simulink model "LQG_Con_lac_nguoc"  (R2023a)
settings: Solver=FixedStepAuto  StartTime=0.0  StopTime=6  FixedStep=0.01  RelTol=1e-3
values from neighbouring files (symbols this model uses):
  A = [ 0,                                                                                                                                                                                                                                                       1,                                                                                                                                                    ...(+372 chars)    [code tìm ma trận K.m]
  B = [                                                                                                                                                                                                                    0,                                                                                                                                                                                          ...(+28 chars)    [code tìm ma trận K.m]
  C = [1 0 0 0 0 0 ... (first row only)    [code tìm ma trận K.m]
  K = lqr(A,B,Q,R_)    [code tìm ma trận K.m]
  L = lqe(A,G,C,QN,RN)    [code tìm ma trận K.m]
undefined symbols (not defined in the file or in its folder): theta_init, thetadot_init, x_init, xdot_init
settings Model: Creator=nhatm  LastModifiedBy=Admin
settings SolverCC: AlgebraicLoopSolver=TrustRegion
settings DataIOCC: ReturnWorkspaceOutputs=off
settings DebuggingCC: UnconnectedInputMsg=warning  UnconnectedOutputMsg=warning  UnconnectedLineMsg=warning  PregeneratedLibrarySubsystemCodeDiagnostic=none  ArithmeticOperatorsInVariantConditions=warning
settings ModelReferenceCC: EnableRefExpFcnMdlSchedulingChecks=on
settings SFSimCC: CustomCodeUndefinedFunction=UseInterfaceOnly

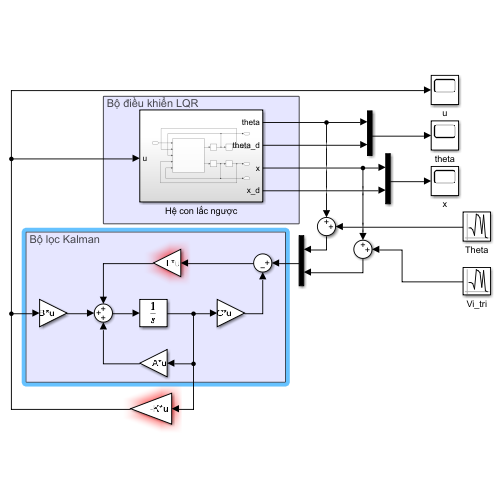
[thumbnail: Simulink's stored preview of the top-level diagram]
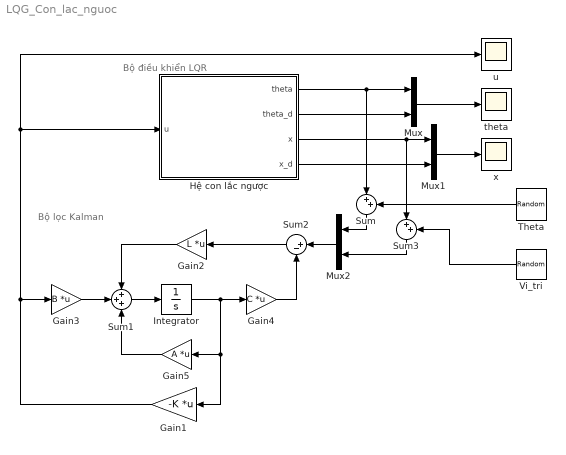
== system LQG_Con_lac_nguoc ==
  note: Bộ lọc Kalman
  note: Bộ điều khiển LQR
  Gain1 : Gain  Gain=-K  Multiplication=Matrix(K*u)
  Gain2 : Gain  Gain=L  Multiplication=Matrix(K*u)
  Gain3 : Gain  Gain=B  Multiplication=Matrix(K*u)
  Gain4 : Gain  Gain=C  Multiplication=Matrix(K*u)
  Gain5 : Gain  Gain=A  Multiplication=Matrix(K*u)
  Hệ con lắc ngược : Subsystem
  Integrator : Integrator
  Mux : Mux  Inputs=2
  Mux1 : Mux  Inputs=2
  Mux2 : Mux  Inputs=2
  Sum : Sum  Inputs=|++
  Sum1 : Sum  Inputs=+++
  Sum2 : Sum  Inputs=|+-
  Sum3 : Sum  Inputs=|++
  Theta : RandomNumber  Variance=0.001  SampleTime=0.01
  Vi_tri : RandomNumber  Variance=0.01  SampleTime=0.01
  theta : Scope
  u : Scope
  x : Scope
  wires:
  Hệ con lắc ngược/1(theta) -> Sum/1, Mux/1
  Hệ con lắc ngược/2(theta_d) -> Mux/2
  Hệ con lắc ngược/3(x) -> Sum3/1, Mux1/1
  Hệ con lắc ngược/4(x_d) -> Mux1/2
  Mux/1 -> theta/1
  Mux1/1 -> x/1
  Sum2/1 -> Gain2/1
  Integrator/1 -> Gain1/1, Gain5/1, Gain4/1
  Sum1/1 -> Integrator/1
  Gain2/1 -> Sum1/1
  Gain5/1 -> Sum1/3
  Gain3/1 -> Sum1/2
  Gain4/1 -> Sum2/2
  Mux2/1 -> Sum2/1
  Gain1/1 -> u/1, Hệ con lắc ngược/1(u), Gain3/1
  Sum/1 -> Mux2/1
  Sum3/1 -> Mux2/2
  Theta/1 -> Sum/2
  Vi_tri/1 -> Sum3/2

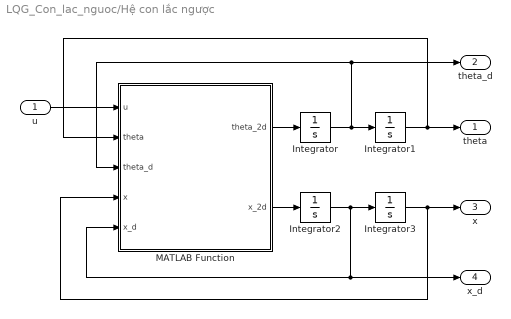
== system LQG_Con_lac_nguoc/Hệ con lắc ngược ==
  u : Inport
  Integrator : Integrator  InitialCondition=thetadot_init
  Integrator1 : Integrator  InitialCondition=theta_init
  Integrator2 : Integrator  InitialCondition=xdot_init
  Integrator3 : Integrator  InitialCondition=x_init
  MATLAB Function : MATLAB Function  TreatAsAtomicUnit=on
  theta : Outport  VectorParamsAs1DForOutWhenUnconnected=off
  theta_d : Outport  Port=2  VectorParamsAs1DForOutWhenUnconnected=off
  x : Outport  Port=3  VectorParamsAs1DForOutWhenUnconnected=off
  x_d : Outport  Port=4  VectorParamsAs1DForOutWhenUnconnected=off
  wires:
  Integrator3/1 -> x/1, MATLAB Function/4(x)
  Integrator/1 -> MATLAB Function/3(theta_d), theta_d/1, Integrator1/1
  MATLAB Function/1(theta_2d) -> Integrator/1
  u/1 -> MATLAB Function/1(u)
  Integrator1/1 -> theta/1, MATLAB Function/2(theta)
  Integrator2/1 -> MATLAB Function/5(x_d), x_d/1, Integrator3/1
  MATLAB Function/2(x_2d) -> Integrator2/1

== matlab function LQG_Con_lac_nguoc/Hệ con lắc ngược/MATLAB Function ==
  data: theta_2d output; u input; x_2d output; theta input; theta_d input; x input; x_d input
function [theta_2d,x_2d] = Inverted_Pendulum(u,theta,theta_d,x,x_d)
M = 1;
m = 0.1;
l = 1;
g = 9.81; %m/s^2
%% Con lac nguoc tren xe
x_2d = (u+m*l*sin(theta)*(theta_d)^2-m*g*cos(theta)*sin(theta))/(M+m-m*(cos(theta))^2);
theta_2d = (u*cos(theta)-(M+m)*g*sin(theta)+m*l*cos(theta)*sin(theta)*(theta_d)^2)/(m*l*(cos(theta))^2-(M+m)*l);
